simulink model "Ice"  (R2020b)
settings: configuration reference "gen_config" (kept outside this file)
undefined symbols (not defined in the file): Ice_derfacLoadDecrease_MAP, Ice_derfacLoadIncrease_MAP, Ice_Load2TqOptIgnLamOne_MAP, Ice_relLoad_AXIS, Ice_relLoad_LoadDyn_AXIS, Ice_relLoad_Max_CUR, Ice_rpm_AXIS, Ice_rpm_LoadDyn_AXIS, Ice_tqLossesIce_MAP
settings Model: DataDictionary=Hybrid_vehicle_update.sldd  SimulationMode=accelerator  Creator=Georg  LastModifiedBy=jy
settings ConfigSetRef: SourceName=gen_config

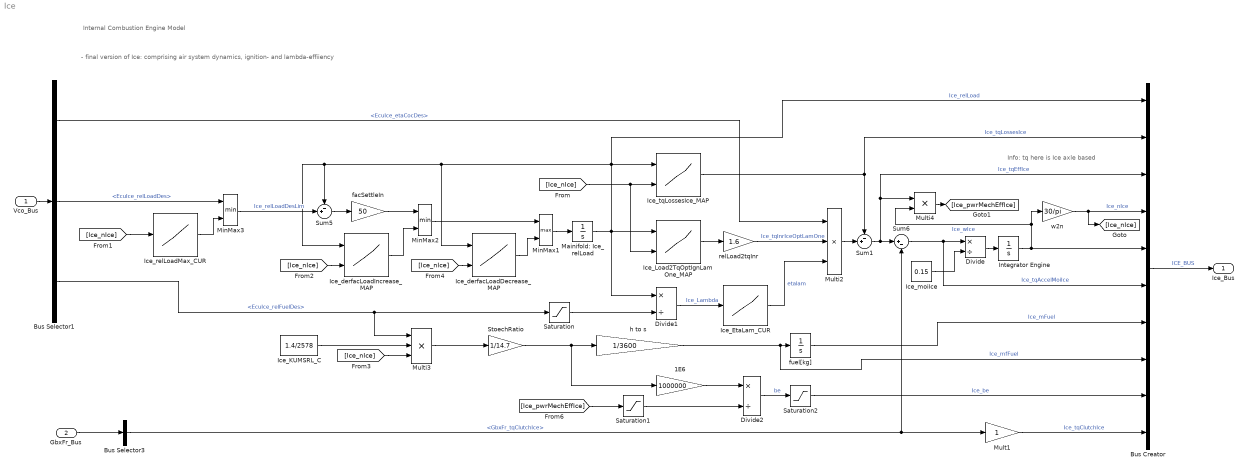
== system Ice ==
  note: Internal Combustion Engine Model
  note: - final version of Ice: comprising air system dynamics, ignition- and lambda-effiiency
  note: Info:
      | tq here is Ice axle based
  Vco_Bus : Inport  OutDataTypeStr=Bus: VCO_BUS
  GbxFr_Bus : Inport  Port=2  OutDataTypeStr=Bus: GBXFR_BUS
  " h to s" : Gain  Gain=1/3600
  1E6 : Gain  Gain=1000000
  Bus Creator : BusCreator  Inputs=10  OutDataTypeStr=Bus: ICE_BUS  NonVirtualBus=on
  Bus Selector1 : BusSelector  OutputSignals=EcuIce_Bus.EcuIce_etaCocDes,EcuIce_Bus.EcuIce_relLoadDes,EcuIce_Bus.EcuIce_relFuelDes
  Bus Selector3 : BusSelector  OutputSignals=GbxFr_tqClutchIce
  Divide : Product  Inputs=*/
  Divide1 : Product  Inputs=*/
  Divide2 : Product  Inputs=*/
  Ice_EtaLam_CUR : Lookup_n-D  NumberOfTableDimensions=1  BreakpointsForDimension1="[0.5    0.6     0.7   0.8   0.85   0.9   1.0   1.1    1.2    1.3    1.4    1.5    1.6    1.7    1.8    1.9    2.0]"  Table="[0       0.5       1     1.1  1.12  1.06   1.0  0.93  0.85   0.78   0.72    0.66    0.625   0.588  0.3  0.2  0]"  ExtrapMethod=Clip  InternalRulePriority=Speed  RndMeth=Simplest  InputSameDT=on
  Ice_KUMSRL_C : Constant  Value=1.4/2578
  Ice_Load2TqOptIgnLamOne_MAP : Lookup_n-D  BreakpointsForDimension1=Ice_relLoad_AXIS  BreakpointsForDimension2=Ice_rpm_AXIS  Table=Ice_Load2TqOptIgnLamOne_MAP  ExtrapMethod=Clip  InternalRulePriority=Speed  RndMeth=Simplest  InputSameDT=on
      settings: InputPortMap=u0,u1
  Ice_derfacLoadDecrease_MAP : Lookup_n-D  BreakpointsForDimension1=Ice_relLoad_LoadDyn_AXIS  BreakpointsForDimension2=Ice_rpm_LoadDyn_AXIS  Table=Ice_derfacLoadDecrease_MAP  ExtrapMethod=Clip  UseLastTableValue=on  InternalRulePriority=Speed  RndMeth=Simplest  InputSameDT=on
      settings: InputPortMap=u0,u1
  Ice_derfacLoadIncrease_MAP : Lookup_n-D  BreakpointsForDimension1=Ice_relLoad_LoadDyn_AXIS  BreakpointsForDimension2=Ice_rpm_LoadDyn_AXIS  Table=Ice_derfacLoadIncrease_MAP  ExtrapMethod=Clip  UseLastTableValue=on  InternalRulePriority=Speed  RndMeth=Simplest  InputSameDT=on
      settings: InputPortMap=u0,u1
  Ice_moiIce : Constant  Value=0.15
  Ice_relLoadMax_CUR : Lookup_n-D  NumberOfTableDimensions=1  BreakpointsForDimension1=Ice_rpm_LoadDyn_AXIS  Table=Ice_relLoad_Max_CUR  ExtrapMethod=Clip  InternalRulePriority=Speed  RndMeth=Simplest  InputSameDT=on
  Ice_tqLossesIce_MAP : Lookup_n-D  BreakpointsForDimension1=Ice_relLoad_AXIS  BreakpointsForDimension2=Ice_rpm_AXIS  Table=Ice_tqLossesIce_MAP  ExtrapMethod=Clip  InternalRulePriority=Speed  RndMeth=Simplest  InputSameDT=on
      settings: InputPortMap=u0,u1
  Integrator Engine : Integrator  LimitOutput=on  LowerSaturationLimit=0
  Mainifold: Ice_relLoad : Integrator  InitialCondition=80  LimitOutput=on  LowerSaturationLimit=0
  MinMax1 : MinMax  Function=max  Inputs=2
  MinMax2 : MinMax  Inputs=2
  MinMax3 : MinMax  Inputs=2
  Mult1 : Gain
  Multi2 : Product  Inputs=***
  Multi3 : Product  Inputs=***
  Multi4 : Product  Inputs=**
  Saturation : Saturate  UpperLimit=1000  LowerLimit=0.0001
  Saturation1 : Saturate  UpperLimit=10000000  LowerLimit=0.1
  Saturation2 : Saturate  UpperLimit=1000  LowerLimit=0
  StoechRatio : Gain  Gain=1/14.7
  Sum1 : Sum  Inputs=-+|
  Sum5 : Sum  Inputs=-+|
  Sum6 : Sum  Inputs=|+-
  facSettleIn : Gain  Gain=50
  fuel[kg] : Integrator
  relLoad2tqInr : Gain  Gain=1.6
  w2n : Gain  Gain=30/pi
  Ice_Bus : Outport  OutDataTypeStr=Bus: ICE_BUS  VectorParamsAs1DForOutWhenUnconnected=off
  wires:
  Sum6/1 -> Bus Creator/6, Divide/1  "Ice_tqAccelMoiIce"
  Mult1/1 -> Bus Creator/10  "Ice_tqClutchIce"
  Multi2/1 -> Sum1/2
  Ice_tqLossesIce_MAP/1 -> Sum1/1, Bus Creator/2  "Ice_tqLossesIce"
  1E6/1 -> Divide2/1
  [Ice_pwrMechEffIce] -> Saturation1/1
  Multi4/1 -> [Ice_pwrMechEffIce]
  Saturation2/1 -> Bus Creator/9  "Ice_be"
  [Ice_nIce] -> Ice_derfacLoadIncrease_MAP/2
  Divide/1 -> Integrator Engine/1
  Saturation1/1 -> Divide2/2
  [Ice_nIce] -> Ice_relLoadMax_CUR/1
  MinMax2/1 -> MinMax1/1
  MinMax1/1 -> Mainifold: Ice_relLoad/1
  " h to s"/1 -> Bus Creator/8, fuel[kg]/1  "Ice_mfFuel"
  StoechRatio/1 -> 1E6/1, " h to s"/1
  Ice_derfacLoadIncrease_MAP/1 -> MinMax2/2
  Ice_EtaLam_CUR/1 -> Multi2/3  "etalam"
  Ice_derfacLoadDecrease_MAP/1 -> MinMax1/2
  Divide2/1 -> Saturation2/1  "be"
  Bus Selector1/1 -> Multi2/1  "<EcuIce_etaCocDes>"
  Saturation/1 -> Divide1/2
  fuel[kg]/1 -> Bus Creator/7  "Ice_mFuel"
  w2n/1 -> Bus Creator/4, [Ice_nIce]  "Ice_nIce"
  Divide1/1 -> Ice_EtaLam_CUR/1  "Ice_Lambda"
  Sum1/1 -> Bus Creator/3, Multi4/1, Sum6/1  "Ice_tqEffIce"
  Bus Selector1/3 -> Multi3/1, Saturation/1  "<EcuIce_relFuelDes>"
  [Ice_nIce] -> Multi3/3
  Bus Selector1/2 -> MinMax3/1  "<EcuIce_relLoadDes>"
  facSettleIn/1 -> MinMax2/1
  [Ice_nIce] -> Ice_Load2TqOptIgnLamOne_MAP/2, Ice_tqLossesIce_MAP/2
  Ice_Load2TqOptIgnLamOne_MAP/1 -> relLoad2tqInr/1
  MinMax3/1 -> Sum5/2  "Ice_relLoadDesLim"
  Multi3/1 -> StoechRatio/1
  relLoad2tqInr/1 -> Multi2/2  "Ice_tqInrIceOptLamOne"
  GbxFr_Bus/1 -> Bus Selector3/1
  Bus Selector3/1 -> Mult1/1, Sum6/2  "<GbxFr_tqClutchIce>"
  Ice_KUMSRL_C/1 -> Multi3/2
  Mainifold: Ice_relLoad/1 -> Divide1/1, Bus Creator/1, Ice_derfacLoadIncrease_MAP/1, Sum5/1, Ice_derfacLoadDecrease_MAP/1, Ice_tqLossesIce_MAP/1, Ice_Load2TqOptIgnLamOne_MAP/1  "Ice_relLoad"
  Sum5/1 -> facSettleIn/1
  Ice_relLoadMax_CUR/1 -> MinMax3/2
  Ice_moiIce/1 -> Divide/2
  [Ice_nIce] -> Ice_derfacLoadDecrease_MAP/2
  Integrator Engine/1 -> Bus Creator/5, w2n/1, Multi4/2  "Ice_wIce"
  Vco_Bus/1 -> Bus Selector1/1
  Bus Creator/1 -> Ice_Bus/1  "ICE_BUS"
